simulink model "power_circ2ss_sps"  (Simulink 6.0)
settings: Solver=ode23tb  SolverMode=SingleTasking  StartTime=0.0  StopTime=0.2  RelTol=1e-3  AbsTol=1e-6
libraries: powerlib x20
settings Model: Creator=patrice  LastModifiedBy=batserve  ExtModeTrigMode=oneshot  ExtModeArmWhenConnect=off  ExtModeAutoUpdateStatusClock=off
settings DataIOCC: LimitDataPoints=off  SignalLoggingName=sigsOut
settings OptimizationCC: BlockReduction=off  BooleanDataType=off
settings DebuggingCC: SolverPrmCheckMsg=none  UnconnectedLineMsg=none
settings HardwareCC: TargetUnknown=on

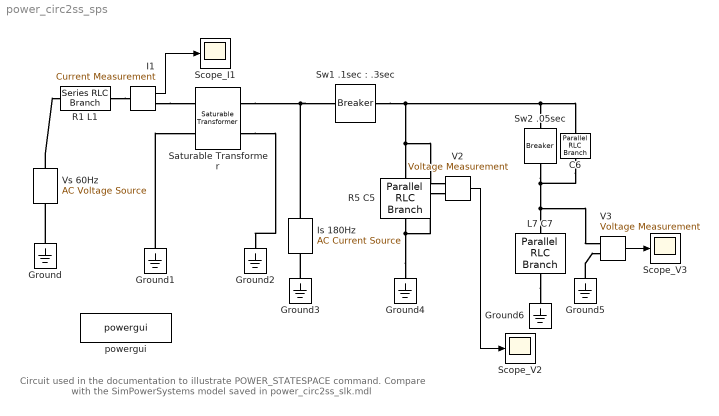
== system power_circ2ss_sps ==
  note: Circuit used in the documentation to illustrate POWER_STATESPACE command.
      | Compare with the SimPowerSystems model saved in power_circ2ss_slk.mdl
  C6 : powerlib/Elements/Parallel RLC Branch  Orientation=down  PhysicalDomain=powersysdomain  SubClassName=unknown  LeftPortType=p1  RightPortType=p1  LConnTagsString=a  RConnTagsString=__new0  Resistance=inf  Inductance=inf  Capacitance=1e-09  Measurements=None
  Ground{,1..6} (7 alike) : powerlib/Elements/Ground  Orientation=down  PhysicalDomain=powersysdomain  SubClassName=unknown  LeftPortType=p1  RightPortType=p1  LConnTagsString=a
  I1 : powerlib/Measurements/Current Measurement  Tag=PoWeRsYsTeMmEaSuReMeNt  PhasorSimulation=off  OutputType=Magnitude  PSBequivalent=0
  Is 180Hz : powerlib/Electrical Sources/AC Current Source  Orientation=up  Amplitude=2  Phase=-30  Frequency=180  SampleTime=0  Measurements=None
      settings: AttributesFormatString=\n
  L7 C7 : powerlib/Elements/Parallel RLC Branch  Orientation=down  PhysicalDomain=powersysdomain  SubClassName=unknown  LeftPortType=p1  RightPortType=p1  LConnTagsString=a  RConnTagsString=__new0  Resistance=inf  Inductance=0.5  Capacitance=2e-06  Measurements=None
  R1 L1 : powerlib/Elements/Series RLC Branch  PhysicalDomain=powersysdomain  SubClassName=unknown  LeftPortType=p1  RightPortType=p1  LConnTagsString=__new0  RConnTagsString=__new0  Resistance=0.1  Inductance=1e-03  Capacitance=inf  Measurements=None
  R5 C5 : powerlib/Elements/Parallel RLC Branch  Orientation=down  PhysicalDomain=powersysdomain  SubClassName=unknown  LeftPortType=p1  RightPortType=p1  LConnTagsString=a  RConnTagsString=__new0  Resistance=200  Inductance=inf  Capacitance=1e-06  Measurements=None
  Saturable Transformer : powerlib/Elements/Saturable Transformer  NominalPower=[10000 60]  Winding1=[100 0.05 1.5e-3*377]  Winding2=[200 0.05 0]  ThreeWindings=off  Winding3=[200 0.05 0]  Saturation=[0 0 ; 0.001 1.2 ; 1 1.3]  CoreLoss=[1000]  Hysteresis=off  DataFile='hysteresis'  Measurements=None  InitialFlux=0  TransfoNumber=1
      settings: AttributesFormatString=\n
  Scope_I1 : Scope
      settings: TickLabels=on  TimeRange=0.2  YMin=-15  YMax=10  DataFormat=Array
  Scope_V2 : Scope
      settings: TickLabels=on  YMin=-200  YMax=200  DataFormat=Array
  Scope_V3 : Scope
      settings: TickLabels=on  TimeRange=0.2  YMin=-400  YMax=400  DataFormat=Array
  "Sw1 .1sec : .3sec" : powerlib/Elements/Breaker  BreakerResistance=0.01  InitialState=1  SnubberResistance=inf  SnubberCapacitance=0  SwitchingTimes="[ .1  .13 ]"  External=off  Measurements=None
      settings: AttributesFormatString=\n
  Sw2 .05sec : powerlib/Elements/Breaker  Orientation=down  BreakerResistance=0.1  InitialState=0  SnubberResistance=inf  SnubberCapacitance=0  SwitchingTimes=[ .05 ]  External=off  Measurements=None
      settings: AttributesFormatString=\n
  V2 : powerlib/Measurements/Voltage Measurement  Tag=PoWeRsYsTeMmEaSuReMeNt  PhasorSimulation=off  OutputType=Magnitude  PSBequivalent=0
  V3 : powerlib/Measurements/Voltage Measurement  Tag=PoWeRsYsTeMmEaSuReMeNt  PhasorSimulation=off  OutputType=Magnitude  PSBequivalent=0
  Vs 60Hz : powerlib/Electrical Sources/AC Voltage Source  Description=source block  Orientation=up  Amplitude=100  Phase=0  Frequency=60  SampleTime=0  Measurements=None
      settings: AttributesFormatString=\n
  powergui : powerlib/powergui  Priority=2  Frange=logspace(0,3,50)  Ylog=off  Xlog=off  save=off  variable=ZData  ZoomFFT=on  StartTime=0.0  cycles=1  DisplayStyle=off  fundamental=60  FreqAxis=off  MaxFrequency=1000  frequencyindice=1  frequencyindicesteady=1  RmsSteady=1  display=off  Ts=0  methode=off  frequency=60  echomessages=off
  wires:
  I1/1 -> Scope_I1/1
  V3/1 -> Scope_V3/1
  V2/1 -> Scope_V2/1
  connections:
  Vs 60Hz/RConn1 -- R1 L1/LConn1
  Ground/LConn1 -- Vs 60Hz/LConn1
  Saturable Transformer/RConn2 -- Ground2/LConn1
  Ground1/LConn1 -- Saturable Transformer/LConn2
  Saturable Transformer/RConn1 -- "Sw1 .1sec : .3sec"/LConn1 -- Is 180Hz/RConn1
  R1 L1/RConn1 -- I1/LConn1
  I1/RConn1 -- Saturable Transformer/LConn1
  Sw2 .05sec/RConn1 -- C6/RConn1 -- L7 C7/LConn1 -- V3/LConn1
  Ground5/LConn1 -- V3/LConn2
  Ground4/LConn1 -- R5 C5/RConn1 -- V2/LConn2
  "Sw1 .1sec : .3sec"/RConn1 -- R5 C5/LConn1 -- V2/LConn1 -- Sw2 .05sec/LConn1 -- C6/LConn1
  Ground3/LConn1 -- Is 180Hz/LConn1
  L7 C7/RConn1 -- Ground6/LConn1
